simulink library "CTC_lib"  (Simulink 7.4)
settings: Solver=ode45  StartTime=0.0  StopTime=10.0  RelTol=1e-3
values from neighbouring files (symbols this model uses):
  CTCc_cnt_PrecGradVoltDeb = mpt.Parameter    [CTC_CAL.m]
  CTCc_i_HVCnctCur_max = mpt.Parameter    [CTC_CAL.m]
  CTCc_i_HVDcnctCur_max = mpt.Parameter    [CTC_CAL.m]
  CTCc_i_HVDcncWaitCur_max = mpt.Parameter    [CTC_CAL.m]
  CTCc_i_PrecCur_max = mpt.Parameter    [CTC_CAL.m]
  CTCc_pct_HVCnctTarVolt = mpt.Parameter    [CTC_CAL.m]
  CTCc_pct_HVDcnctTarVolt = mpt.Parameter    [CTC_CAL.m]
  CTCc_pct_NegCtrDiagCld = mpt.Parameter    [CTC_CAL.m]
  CTCc_pct_NegCtrDiagOpen = mpt.Parameter    [CTC_CAL.m]
  CTCc_pct_PosCtrDiagCld = mpt.Parameter    [CTC_CAL.m]
  CTCc_pct_PosCtrDiagOpen = mpt.Parameter    [CTC_CAL.m]
  CTCc_pct_PrecTarVolt = mpt.Parameter    [CTC_CAL.m]
  CTCc_pct_PrecVoltAllow = mpt.Parameter    [CTC_CAL.m]
  CTCc_tm_CtrClsCheckDly = mpt.Parameter    [CTC_CAL.m]
  CTCc_tm_CtrClsCheckDly_max = mpt.Parameter    [CTC_CAL.m]
  CTCc_tm_CtrOpenCheck_max = mpt.Parameter    [CTC_CAL.m]
  CTCc_tm_CtrOpenCheckDly = mpt.Parameter    [CTC_CAL.m]
  CTCc_tm_HVCnctTm_max = mpt.Parameter    [CTC_CAL.m]
  CTCc_tm_HVDcnctTm_max = mpt.Parameter    [CTC_CAL.m]
  CTCc_tm_HVDcnctWaitTm = mpt.Parameter    [CTC_CAL.m]
  CTCc_tm_HVDcnctWaitTm_max = mpt.Parameter    [CTC_CAL.m]
  CTCc_tm_HVEmcyDcnctTm_max = mpt.Parameter    [CTC_CAL.m]
  CTCc_tm_PrecTm_max = mpt.Parameter    [CTC_CAL.m]
  CTCc_tm_PrecVoltAlow = mpt.Parameter    [CTC_CAL.m]
  CTCc_tm_Tick_s = mpt.Parameter    [CTC_CAL.m]
  CTCc_v_PrecGradVolt = mpt.Parameter    [CTC_CAL.m]
  CTCc_v_PrecTarVoltDif = mpt.Parameter    [CTC_CAL.m]
libraries: Defined_Functionality x4
(part 2 of 2)

== stateflow chart CTC/ContactorControl ==
  settings: sampleTime=0.01
  settings: description=|
      | $Author:Zhao XiangRi$
      | $Date:2015/03/26$
      | $Revision:1.0$
  state Timer [function]
    state T1 [function]
      settings: description=$Author:Zhao XiangRi$
      state Run(Limit) [function]
        settings: description=$Author:Zhao XiangRi$
        (default) -> (junction 185)
        (junction 185) -> (junction 186) [order 1] : [Init != 1]
            | {TimeTicks = 0;TimeLimit = Limit / 10;Init = 1;}
        (junction 186) -> (junction 185)
        (junction 185) -> (junction 187) [order 2] : {TimeTicks++;}
        (junction 187) -> (junction 188) [order 1] : [TimeTicks >= TimeLimit]{Timeout = 1;}
        (junction 187) -> (junction 189) [order 2]
      state Clear [function]
        settings: description=$Author:Zhao XiangRi$
        (default) -> (junction 190)
        (junction 190) -> (junction 191) : {Timeout = 0;Init = 0;}
    state T2 [function]
      settings: description=$Author:Zhao XiangRi$
      state Run(Limit) [function]
        settings: description=$Author:Zhao XiangRi$
        (default) -> (junction 192)
        (junction 192) -> (junction 193) [order 1] : [Init != 1]{TimeTicks = 0;TimeLimit = Limit / 10;Init = 1;}
        (junction 193) -> (junction 192)
        (junction 192) -> (junction 194) [order 2] : {TimeTicks++;}
        (junction 194) -> (junction 195) [order 1] : [TimeTicks >= TimeLimit]{Timeout = 1;}
        (junction 194) -> (junction 196) [order 2]
      state Clear [function]
        settings: description=$Author:Zhao XiangRi$
        (default) -> (junction 197)
        (junction 197) -> (junction 198) : {Timeout = 0;
            | Init = 0;}
    state T3 [function]
      settings: description=$Author:Zhao XiangRi$
      state Run(Limit) [function]
        settings: description=$Author:Zhao XiangRi$
        (default) -> (junction 199)
        (junction 199) -> (junction 200) [order 1] : [Init != 1]{TimeTicks = 0;TimeLimit = Limit / 10;Init = 1;}
        (junction 200) -> (junction 199)
        (junction 199) -> (junction 201) [order 2] : {TimeTicks++;}
        (junction 201) -> (junction 202) [order 1] : [TimeTicks >= TimeLimit]{Timeout = 1;}
        (junction 201) -> (junction 203) [order 2]
      state Clear [function]
        settings: description=$Author:Zhao XiangRi$
        (default) -> (junction 204)
        (junction 204) -> (junction 205) : {Timeout = 0;Init = 0;}
    state T4 [function]
      settings: description=$Author:Zhao XiangRi$
      state Run(Limit) [function]
        settings: description=$Author:Zhao XiangRi$
        (default) -> (junction 206)
        (junction 206) -> (junction 207) [order 1] : [Init != 1]{TimeTicks = 0;TimeLimit = Limit / 10;Init = 1;}
        (junction 207) -> (junction 206)
        (junction 206) -> (junction 208) [order 2] : {TimeTicks++;}
        (junction 208) -> (junction 209) [order 1] : [TimeTicks >= TimeLimit]{Timeout = 1;}
        (junction 208) -> (junction 210) [order 2]
      state Clear [function]
        settings: description=$Author:Zhao XiangRi$
        (default) -> (junction 211)
        (junction 211) -> (junction 212) : {Timeout = 0;Init = 0;}
  state FastCharge
    settings: description=|
        | $Author:Zhao XiangRi$
        | $Date:2015/03/25$
        | $Revision:1.0$
    state FastChaCtrConnect
      en:
      CTCd_enum_CtrSt = CTC_FastChaConnect_St;
      FastChaConnectFinish=0;
      settings: description=$Author:Zhao XiangRi$
      state FastChaContactorControl
        en:
        CTCd_flg_FastChaCtrSt=0;
        ex:
        Timer.T1.Clear();
        state CloseFastChaContactorFinish
          en:
          CTCd_flg_FastChaCtrSt=1;
        state CloseFastChaContactor
          en:
          CTCd_flg_FastChaCtrReq= 1;
          du:
          Timer.T1.Run(CTCc_tm_CtrClsCheckDly);
          ex:
          Timer.T1.Clear();
        CloseFastChaContactor -> CloseFastChaContactorFinish : [Timer.T1.Timeout==1]
        (default) -> CloseFastChaContactor
      state FastChaConnectFinish
        en:
        FastChaConnectFinish=1;
      state NegContactorControl
        en:
        CTCd_flg_NegCtrSt=0;
        ex:
        Timer.T1.Clear();
        Timer.T2.Clear();
        CTCd_iflt_NegCtrStuckOpen_fault=0;
        state CloseNegContactorFinish
          en:
          CTCd_flg_NegCtrSt=1;
          CTCd_iflt_NegCtrStuckOpen_fault=0;
        state CloseNegTimeOut
          en:
          CTCd_iflt_NegCtrStuckOpen_fault=1;
        state CloseNegContactor
          en:
          CTCd_flg_NegCtrReq= 1;
          du:
          Timer.T1.Run(CTCc_tm_CtrClsCheckDly);
          Timer.T2.Run(CTCc_tm_CtrClsCheckDly_max);
        (default) -> FastCharge.FastChaCtrConnect.NegContactorControl.CloseNegContactor
        FastCharge.FastChaCtrConnect.NegContactorControl.CloseNegTimeOut -> FastCharge.FastChaCtrConnect.NegContactorControl.CloseNegContactor
        FastCharge.FastChaCtrConnect.NegContactorControl.CloseNegContactor -> FastCharge.FastChaCtrConnect.NegContactorControl.CloseNegTimeOut [order 1] : [Timer.T2.Timeout==1&&CTCd_iflt_NegCtrStuckOpen_fault!=1]
        FastCharge.FastChaCtrConnect.NegContactorControl.CloseNegContactor -> FastCharge.FastChaCtrConnect.NegContactorControl.CloseNegContactorFinish [order 2] : [UAct3 <= UAct1 *(1+ CTCc_pct_NegCtrDiagCld)&&...
            | UAct3 >= UAct1 *(1- CTCc_pct_NegCtrDiagCld)&&...
            | Timer.T1.Timeout==1]
      (default) -> FastCharge.FastChaCtrConnect.NegContactorControl
      FastCharge.FastChaCtrConnect.NegContactorControl.CloseNegContactorFinish -> FastCharge.FastChaCtrConnect.FastChaContactorControl : [CTCd_flg_NegCtrSt==1]
      CloseFastChaContactorFinish -> FastCharge.FastChaCtrConnect.FastChaConnectFinish : [CTCd_flg_FastChaCtrSt==1]
    state FastChaOffline
      CTCd_enum_CtrSt = CTC_FastChaOffline_St;
      CTCd_flg_NegCtrReq = 0;
      CTCd_flg_FastChaCtrReq = 0;
      CTCd_flg_NegCtrSt = 0;
      CTCd_flg_FastChaCtrSt = 0;
      settings: description=$Author:Zhao XiangRi$
    state FastChaDisconnect
      en:
      CTCd_enum_CtrSt=CTC_FastChaDisconnect_St;
      FastChaDisconnectFinish=0;
      settings: description=$Author:Zhao XiangRi$
      state FastChaContactorControl
        state OpenFastChaContactorFinish
          en:
          CTCd_flg_FastChaCtrSt=0;
        state OpenFastChaContactor
          en:
          CTCd_flg_FastChaCtrReq= 0;
          du:
          Timer.T1.Run(CTCc_tm_CtrOpenCheckDly);
          ex:
          Timer.T1.Clear();
        OpenFastChaContactor -> OpenFastChaContactorFinish : [Timer.T1.Timeout==1]
        (default) -> OpenFastChaContactor
      state FastChaConnectFinish
        en:
        FastChaDisconnectFinish=1;
      state NegContactorControl
        ex:
        CTCd_iflt_NegCtrStuckCld_fault=0;
        state OpenNegTimeOut
          en:
          CTCd_iflt_NegCtrStuckCld_fault=1;
        state OpenPosContactorFinish
          en:
          CTCd_flg_NegCtrSt=0;
          CTCd_iflt_NegCtrStuckCld_fault=0;
        state OpenNegContactor
          en:
          CTCd_flg_NegCtrReq= 0;
          du:
          Timer.T1.Run(CTCc_tm_CtrOpenCheckDly);
          Timer.T2.Run(CTCc_tm_CtrOpenCheck_max);
          ex:
          Timer.T1.Clear();
          Timer.T2.Clear();
        FastCharge.FastChaDisconnect.NegContactorControl.OpenNegTimeOut -> FastCharge.FastChaDisconnect.NegContactorControl.OpenNegContactor
        FastCharge.FastChaDisconnect.NegContactorControl.OpenNegContactor -> FastCharge.FastChaDisconnect.NegContactorControl.OpenPosContactorFinish [order 1] : [Timer.T1.Timeout==1&&(UAct3>= UAct1 * (1 + CTCc_pct_NegCtrDiagOpen) || ...
            | UAct3<= UAct1 * (1 - CTCc_pct_NegCtrDiagOpen))]
        (default) -> FastCharge.FastChaDisconnect.NegContactorControl.OpenNegContactor
        FastCharge.FastChaDisconnect.NegContactorControl.OpenNegContactor -> FastCharge.FastChaDisconnect.NegContactorControl.OpenNegTimeOut [order 2] : [Timer.T2.Timeout==1&&CTCd_iflt_NegCtrStuckCld_fault!=1]
      FastCharge.FastChaDisconnect.NegContactorControl.OpenPosContactorFinish -> FastCharge.FastChaDisconnect.FastChaConnectFinish : [CTCd_flg_NegCtrSt==0]
      (default) -> FastCharge.FastChaDisconnect.FastChaContactorControl
      OpenFastChaContactorFinish -> FastCharge.FastChaDisconnect.NegContactorControl : [CTCd_flg_FastChaCtrSt==0]
    state FastChaCtrOnline
      en:
      CTCd_enum_CtrSt=CTC_FastChaOnline_St;
      settings: description=$Author:Zhao XiangRi$
    (default) -> FastChaOffline
    (junction 240) -> FastChaOffline
    (junction 241) -> (junction 240)
    FastChaCtrOnline -> FastChaDisconnect : [DEMd_enum_CtrCmd==CTC_FastChaOffline_CtrCmd||...
        | DEMd_enum_CtrCmd~=CTC_FastChaOnline_CtrCmd]
    FastChaOffline -> FastChaCtrConnect : [DEMd_enum_CtrCmd==CTC_FastChaOnline_CtrCmd]
    FastCharge.FastChaCtrConnect.FastChaConnectFinish -> FastChaCtrOnline : [FastChaConnectFinish==1]
    FastCharge.FastChaDisconnect.FastChaConnectFinish -> (junction 241) : [FastChaDisconnectFinish==1]
  state Drive
    settings: description=|
        | $Author:Zhao XiangRi$
        | $Date:2015/03/20$
        | $Revision:1.0$
    state Offline
      CTCd_enum_CtrSt = CTC_DriveOffline_St;
      CTCd_flg_PosCtrReq = 0;
      CTCd_flg_NegCtrReq = 0;
      CTCd_flg_PreCtrReq = 0;
      CTCd_flg_PosCtrSt = 0;
      CTCd_flg_NegCtrSt = 0;
      CTCd_flg_PreCtrSt = 0;
      ex:
      Timer.T3.Clear();
      Timer.T4.Clear();
      settings: description=$Author:Zhao XiangRi$
      state PreChargeProhibit
        en:
        PreChargeAllow=0;
        du:
        Timer.T3.Run(CTCc_tm_PrecVoltAlow);
        ex:
        Timer.T3.Clear();
      state PreChargeAllow
        en:
        PreChargeAllow=1;
        du:
        Timer.T4.Run(CTCc_tm_PrecVoltAlow);
        ex:
        Timer.T4.Clear();
      (default) -> Drive.Offline.PreChargeProhibit
      Drive.Offline.PreChargeAllow -> Drive.Offline.PreChargeProhibit [order 1] : [UAct4>= (UAct1 * CTCc_pct_PrecVoltAllow)&&...
          | Timer.T4.Timeout ==1]
      Drive.Offline.PreChargeProhibit -> Drive.Offline.PreChargeAllow : [UAct4<(UAct1 * CTCc_pct_PrecVoltAllow)&&...
          | Timer.T3.Timeout ==1]
    state PreCharge
      en:
      CTCd_enum_CtrSt=CTC_DrivePrecharge_St;
      CTCd_flg_NegCtrSt=0;
      CTCd_flg_PreCtrSt=0;
      PreChargeFinish=0;
      du:
      CurrentGuard();
      ex:
      CTCd_iflt_NegCtrStuckOpen_fault=0;
      CTCd_iflt_PrecCurOver_fault=0;
      CTCd_iflt_PrecTmOver_fault=0;
      settings: description=$Author:Zhao XiangRi$
      state CurrentGuard [function]
        settings: description=$Author:Zhao XiangRi$
        (default) -> (junction 214)
        (junction 214) -> (junction 213) [order 3]
        (junction 214) -> (junction 215) [order 2] : [IAct<= CTCc_i_PrecCur_max && CTCd_iflt_PrecCurOver_fault != 0]
            | {CTCd_iflt_PrecCurOver_fault = 0;}
        (junction 214) -> (junction 216) [order 1] : [IAct>CTCc_i_PrecCur_max&& CTCd_iflt_PrecCurOver_fault!=1]
            | {CTCd_iflt_PrecCurOver_fault=1;}
      state NegContactorControl
        en:
        CTCd_flg_NegCtrSt=0;
        ex:
        Timer.T1.Clear();
        Timer.T2.Clear();
        CTCd_iflt_NegCtrStuckOpen_fault=0;
        settings: description=$Author:Zhao XiangRi$
        state CloseNegContactor
          en:
          CTCd_flg_NegCtrReq= 1;
          du:
          Timer.T1.Run(CTCc_tm_CtrClsCheckDly);
          Timer.T2.Run(CTCc_tm_CtrClsCheckDly_max);
        state CloseNegTimeOut
          en:
          CTCd_iflt_NegCtrStuckOpen_fault=1;
        state CloseNegContactorFinish
          en:
          CTCd_flg_NegCtrSt=1;
          CTCd_iflt_NegCtrStuckOpen_fault=0;
        (default) -> Drive.PreCharge.NegContactorControl.CloseNegContactor
        Drive.PreCharge.NegContactorControl.CloseNegContactor -> Drive.PreCharge.NegContactorControl.CloseNegTimeOut [order 1] : [Timer.T2.Timeout==1&&CTCd_iflt_NegCtrStuckOpen_fault!=1]
        Drive.PreCharge.NegContactorControl.CloseNegTimeOut -> Drive.PreCharge.NegContactorControl.CloseNegContactor
        Drive.PreCharge.NegContactorControl.CloseNegContactor -> Drive.PreCharge.NegContactorControl.CloseNegContactorFinish [order 2] : [UAct3 <= UAct1 *(1+ CTCc_pct_NegCtrDiagCld)&&...
            | UAct3 >= UAct1 *(1- CTCc_pct_NegCtrDiagCld)&&...
            | Timer.T1.Timeout==1]
      state PreContactorControl
        en:
        CTCd_flg_PreCtrSt=0;
        ex:
        Timer.T1.Clear();
        settings: description=$Author:Zhao XiangRi$
        state ClosePreContactor
          en:
          CTCd_flg_PreCtrReq= 1;
          du:
          Timer.T1.Run(CTCc_tm_CtrClsCheckDly);
          ex:
          Timer.T1.Clear();
        state ClosePreContactorFinish
          en:
          CTCd_flg_PreCtrSt=1;
        (default) -> Drive.PreCharge.PreContactorControl.ClosePreContactor
        Drive.PreCharge.PreContactorControl.ClosePreContactor -> Drive.PreCharge.PreContactorControl.ClosePreContactorFinish : [Timer.T1.Timeout==1]
      state PreChargeCheck
        du:
        Timer.T3.Run(CTCc_tm_PrecTm_max);
        ex:
        CTCd_iflt_PrecTmOver_fault= 0;
        Timer.T3.Clear();
        settings: description=$Author:Zhao XiangRi$
        state VoltageGradientCheck [function]
          settings: description=$Author:Zhao XiangRi$
          state Run(GradLimit,CountLimit) [function]
            (default) -> (junction 217)
            (junction 217) -> (junction 218) [order 1] : [GradLimitCorr == 0]
                | {GradLimitCorr = GradLimit * CTCc_tm_Tick_s;}
            (junction 218) -> (junction 217)
            (junction 217) -> (junction 219) [order 2] : {UGrad = UAct2 - UMem;}
            (junction 219) -> (junction 220) : {UMem = UAct2;}
            (junction 222) -> (junction 221) [order 1] : [Count >= CountLimit]
                | {Ok = 1;}
            (junction 220) -> (junction 222) [order 1] : [UGrad * CTCc_tm_Tick_s <= GradLimitCorr]
            (junction 222) -> (junction 223) [order 2] : {Count++;}
            (junction 220) -> (junction 223) [order 2] : {Ok = 0; Count = 0;}
          state Init [function]
            (default) -> (junction 224)
            (junction 224) -> (junction 225) : {UMem = 0; UGrad = 0; Count = 0; Ok = 0;...
                | GradLimitCorr = 0;}
        state PreChargeWait
          en:
          VoltageGradientCheck.Init();
          du:
          VoltageGradientCheck.Run(CTCc_v_PrecGradVolt,CTCc_cnt_PrecGradVoltDeb);
        state PrecDurMaxError
          en:
          CTCd_iflt_PrecTmOver_fault=1;
        state PreChargeFinish
          en:
          PreChargeFinish=1;
          CTCd_iflt_PrecTmOver_fault=0;
        (default) -> Drive.PreCharge.PreChargeCheck.PreChargeWait
        Drive.PreCharge.PreChargeCheck.PreChargeWait -> Drive.PreCharge.PreChargeCheck.PrecDurMaxError [order 2] : [Timer.T3.Timeout ==1 &&CTCd_iflt_PrecTmOver_fault!= 1]
        Drive.PreCharge.PreChargeCheck.PrecDurMaxError -> Drive.PreCharge.PreChargeCheck.PreChargeWait
        Drive.PreCharge.PreChargeCheck.PreChargeWait -> Drive.PreCharge.PreChargeCheck.PreChargeFinish [order 1] : [UAct2>= (UAct1 * CTCc_pct_PrecTarVolt)&&...
            | (UAct1 - UAct2) <= CTCc_v_PrecTarVoltDif&&...
            | VoltageGradientCheck.Ok == 1&&...
            | CTCd_flg_PreCtrSt==1&&CTCd_flg_NegCtrSt==1]
      (default) -> Drive.PreCharge.NegContactorControl
      Drive.PreCharge.NegContactorControl.CloseNegContactorFinish -> Drive.PreCharge.PreContactorControl : [CTCd_flg_NegCtrSt==1]
      Drive.PreCharge.PreContactorControl.ClosePreContactorFinish -> Drive.PreCharge.PreChargeCheck : [CTCd_flg_PreCtrSt==1]
    state Connect
      en:
      CTCd_enum_CtrSt=...
      CTC_DriveConnect_St;
      CTCd_flg_PosCtrSt=0;
      ConnectFinish=0;
      ex:
      CTCd_iflt_HVCnctCurOver_fault = 0;
      CTCd_iflt_HVCnctTmOver_fault=0;
      settings: description=$Author:Zhao XiangRi$
      state ConnectControl [parallel]
        settings: executionOrder=1  description=$Author:Zhao XiangRi$
        state PosContactorControl
          en:
          CTCd_flg_PosCtrSt=0;
          ex:
          CTCd_iflt_PosCtrStuckOpen_fault=0;
          settings: description=$Author:Zhao XiangRi$
          state ClosePosContactor
            en:
            CTCd_flg_PosCtrReq= 1;
            du:
            Timer.T1.Run(CTCc_tm_CtrClsCheckDly);
            Timer.T2.Run(CTCc_tm_CtrClsCheckDly_max);
            ex:
            Timer.T1.Clear();
            Timer.T2.Clear();
          state ClosePosTimeOut
            en:
            CTCd_iflt_PosCtrStuckOpen_fault=1;
          state ClosePosContactorFinish
            en:
            CTCd_flg_PosCtrSt=1;
            CTCd_iflt_PosCtrStuckOpen_fault=0;
          (default) -> Drive.Connect.ConnectControl.PosContactorControl.ClosePosContactor
          Drive.Connect.ConnectControl.PosContactorControl.ClosePosContactor -> Drive.Connect.ConnectControl.PosContactorControl.ClosePosTimeOut [order 1] : [Timer.T2.Timeout==1&&CTCd_iflt_PosCtrStuckOpen_fault!=1]
          Drive.Connect.ConnectControl.PosContactorControl.ClosePosTimeOut -> Drive.Connect.ConnectControl.PosContactorControl.ClosePosContactor
          Drive.Connect.ConnectControl.PosContactorControl.ClosePosContactor -> Drive.Connect.ConnectControl.PosContactorControl.ClosePosContactorFinish [order 2] : [Timer.T1.Timeout==1&&...
              | UAct2<=UAct1 * (1+CTCc_pct_PosCtrDiagCld)&& ...
              | UAct2>= UAct1 *(1-CTCc_pct_PosCtrDiagCld) ]
        state PreContactorControl
          settings: description=$Author:Zhao XiangRi$
          state OpenPreContactor
            en:
            CTCd_flg_PreCtrReq= 0;
            du:
            Timer.T1.Run(CTCc_tm_CtrOpenCheckDly);
            ex:
            Timer.T1.Clear();
          state OpenPosContactorFinish
            en:
            CTCd_flg_PreCtrSt=0;
          (default) -> Drive.Connect.ConnectControl.PreContactorControl.OpenPreContactor
          Drive.Connect.ConnectControl.PreContactorControl.OpenPreContactor -> Drive.Connect.ConnectControl.PreContactorControl.OpenPosContactorFinish : [Timer.T1.Timeout==1]
        (default) -> Drive.Connect.ConnectControl.PosContactorControl
        Drive.Connect.ConnectControl.PosContactorControl.ClosePosContactorFinish -> Drive.Connect.ConnectControl.PreContactorControl : [CTCd_flg_PosCtrSt==1]
      state ConnectCheck [parallel]
        du:
        CurrentGuard();
        Timer.T3.Run(CTCc_tm_HVCnctTm_max);
        ex:
        Timer.T3.Clear();
        settings: executionOrder=2  description=$Author:Zhao XiangRi$
        state CurrentGuard [function]
          settings: description=$Author:Zhao XiangRi$
          (default) -> (junction 227)
          (junction 227) -> (junction 226) [order 3]
          (junction 227) -> (junction 228) [order 2] : [IAct<= CTCc_i_HVCnctCur_max&& CTCd_iflt_HVCnctCurOver_fault != 0]
              | {CTCd_iflt_HVCnctCurOver_fault = 0;}
          (junction 227) -> (junction 229) [order 1] : [IAct> CTCc_i_HVCnctCur_max&& CTCd_iflt_HVCnctCurOver_fault != 1]
              | {CTCd_iflt_HVCnctCurOver_fault = 1;}
        state ConnectWait
        state CnctDurMaxError
          en:
          CTCd_iflt_HVCnctTmOver_fault=1;
        state ConnectFinish
          en:
          ConnectFinish=1;
          CTCd_iflt_HVCnctTmOver_fault=0;
        (default) -> Drive.Connect.ConnectCheck.ConnectWait
        Drive.Connect.ConnectCheck.ConnectWait -> Drive.Connect.ConnectCheck.CnctDurMaxError [order 2] : [Timer.T3.Timeout ==1&&CTCd_iflt_HVCnctTmOver_fault!=1]
        Drive.Connect.ConnectCheck.CnctDurMaxError -> Drive.Connect.ConnectCheck.ConnectWait
        Drive.Connect.ConnectCheck.ConnectWait -> Drive.Connect.ConnectCheck.ConnectFinish [order 1] : [UAct2 >= (UAct1 * CTCc_pct_HVCnctTarVolt)&&...
            |  CTCd_flg_PosCtrSt==1&&...
            | CTCd_flg_PreCtrSt==0]
    state Online
      en:
      CTCd_enum_CtrSt=CTC_DriveOnline_St;
      settings: description=$Author:Zhao XiangRi$
      state NegContactorDiagnose [parallel]
        ex:
        Timer.T1.Clear();
        CTCd_iflt_NegCtrStuckOpen_fault=0;
        settings: executionOrder=1  description=$Author:Zhao XiangRi$
        state NegContactorCheck
          en:
          CTCd_iflt_NegCtrStuckOpen_fault=0;
          Timer.T1.Clear();
        state NegContactorDiag
          du:
          Timer.T1.Run(CTCc_tm_CtrOpenCheck_max);
        state NegContactorFault
          en:
          CTCd_flg_NegCtrSt=0;
          CTCd_iflt_NegCtrStuckOpen_fault=1;
          Timer.T1.Clear();
        (default) -> Drive.Online.NegContactorDiagnose.NegContactorCheck
        Drive.Online.NegContactorDiagnose.NegContactorCheck -> Drive.Online.NegContactorDiagnose.NegContactorDiag : [UAct3 > UAct1 *(1+ CTCc_pct_NegCtrDiagOpen)||...
            | UAct3 < UAct1 *(1- CTCc_pct_NegCtrDiagOpen)]
        Drive.Online.NegContactorDiagnose.NegContactorDiag -> Drive.Online.NegContactorDiagnose.NegContactorCheck [order 1] : [UAct3 < UAct1 *(1+ CTCc_pct_NegCtrDiagCld)&&...
            | UAct3 >UAct1 *(1- CTCc_pct_NegCtrDiagCld)]
        Drive.Online.NegContactorDiagnose.NegContactorDiag -> Drive.Online.NegContactorDiagnose.NegContactorFault [order 2] : [(UAct3 > UAct1 *(1+ CTCc_pct_NegCtrDiagOpen)||...
            | UAct3 < UAct1 *(1- CTCc_pct_NegCtrDiagOpen))&&...
            | (CTCd_iflt_NegCtrStuckOpen_fault!=1)&&...
            | Timer.T1.Timeout==1]
      state PosContactorDiagnose [parallel]
        ex:
        Timer.T2.Clear();
        CTCd_iflt_PosCtrStuckOpen_fault=0;
        settings: executionOrder=2  description=$Author:Zhao XiangRi$
        state PosContactorDiag
          du:
          Timer.T2.Run(CTCc_tm_CtrOpenCheck_max);
        state PosContactorCheck
          en:
          CTCd_iflt_PosCtrStuckOpen_fault=0;
          Timer.T2.Clear();
        state PosContactorFault
          en:
          CTCd_flg_PosCtrSt=0;
          CTCd_iflt_PosCtrStuckOpen_fault=1;
          Timer.T2.Clear();
        (default) -> Drive.Online.PosContactorDiagnose.PosContactorCheck
        Drive.Online.PosContactorDiagnose.PosContactorCheck -> Drive.Online.PosContactorDiagnose.PosContactorDiag : [UAct2 > UAct1 *(1+ CTCc_pct_PosCtrDiagOpen)||...
            | UAct2 < UAct1 *(1- CTCc_pct_PosCtrDiagOpen)]
        Drive.Online.PosContactorDiagnose.PosContactorDiag -> Drive.Online.PosContactorDiagnose.PosContactorCheck [order 1] : [UAct2<UAct1 *(1+ CTCc_pct_PosCtrDiagCld)&&...
            | UAct2>UAct1 *(1- CTCc_pct_PosCtrDiagCld)]
        Drive.Online.PosContactorDiagnose.PosContactorDiag -> Drive.Online.PosContactorDiagnose.PosContactorFault [order 2] : [(UAct2 > UAct1 *(1+ CTCc_pct_PosCtrDiagOpen)||...
            | UAct2 < UAct1 *(1- CTCc_pct_PosCtrDiagOpen))&&...
            | CTCd_iflt_PosCtrStuckOpen_fault!=1&&...
            | Timer.T2.Timeout==1]
    state EmergencyDisconnect
      en:
      CTCd_enum_CtrSt=...
      CTC_DriveEmgyDcnct_St;
      DcnctEmcyFinish = 0;
      settings: description=$Author:Zhao XiangRi$
      state EmcyDisconnectControl [parallel]
        en:
        CTCd_flg_PosCtrReq= 0;
        CTCd_flg_NegCtrReq= 0;
        CTCd_flg_PreCtrReq= 0;
        DcnctEmcyCtlFinish = 1;
        settings: executionOrder=1  description=$Author:Zhao XiangRi$
      state EmcyDisconnectCheck [parallel]
        du:
        Timer.T1.Run(CTCc_tm_HVEmcyDcnctTm_max);
        ex:
        Timer.T1.Clear();
        settings: executionOrder=2  description=$Author:Zhao XiangRi$
        state DisconnectWait
        state DisconnectComplete
          DcnctEmcyFinish = 1;
        state DisconnectTimeoutError
          en:
          CTCd_iflt_HVEmcyDcnctTmOver_fault = 1;
          ex:
          CTCd_iflt_HVEmcyDcnctTmOver_fault = 0;
        (default) -> Drive.EmergencyDisconnect.EmcyDisconnectCheck.DisconnectWait
        Drive.EmergencyDisconnect.EmcyDisconnectCheck.DisconnectWait -> Drive.EmergencyDisconnect.EmcyDisconnectCheck.DisconnectComplete [order 2] : [DcnctEmcyCtlFinish==1 &&IAct<= CTCc_i_HVDcnctCur_max &&...
            | (UAct2>= UAct1 * (1 + CTCc_pct_HVDcnctTarVolt) ||UAct2<= UAct1 * (1 - CTCc_pct_HVDcnctTarVolt))]
            | {CTCd_flg_PosCtrSt=0;CTCd_flg_NegCtrSt=0;CTCd_flg_PreCtrSt=0;}
        Drive.EmergencyDisconnect.EmcyDisconnectCheck.DisconnectWait -> Drive.EmergencyDisconnect.EmcyDisconnectCheck.DisconnectTimeoutError [order 1] : [Timer.T1.Timeout == 1]
        Drive.EmergencyDisconnect.EmcyDisconnectCheck.DisconnectTimeoutError -> Drive.EmergencyDisconnect.EmcyDisconnectCheck.DisconnectComplete : [DcnctEmcyCtlFinish==1 &&...
            | (UAct2>= UAct1 * (1 +CTCc_pct_HVDcnctTarVolt) ||UAct2<= UAct1 * (1 - CTCc_pct_HVDcnctTarVolt))]
            | {CTCd_flg_PosCtrSt=0;CTCd_flg_NegCtrSt=0;CTCd_flg_PreCtrSt=0;}
    state Shutoff
      en:
      CTCd_enum_CtrSt=CTC_DriveShutoff_St;
      ShutoffFinish=0;
      ex:
      CTCd_iflt_HVDcncWaitTmOver_fault=0;
      Timer.T1.Clear();
      Timer.T2.Clear();
      settings: description=$Author:Zhao XiangRi$
      state ShutoffDelay
        en:
        ShutoffFinish = 0;
        du:
        Timer.T1.Run(CTCc_tm_HVDcnctWaitTm_max);
        Timer.T2.Run(CTCc_tm_HVDcnctWaitTm);
      state SoffDurMaxError
        en:
        CTCd_iflt_HVDcncWaitTmOver_fault = 1;
      state ShutoffComplete
        en:
        ShutoffFinish=1;
        CTCd_iflt_HVDcncWaitTmOver_fault = 0;
      (default) -> ShutoffDelay
      ShutoffDelay -> SoffDurMaxError [order 2] : [Timer.T1.Timeout == 1 && CTCd_iflt_HVDcncWaitTmOver_fault != 1]
      SoffDurMaxError -> ShutoffDelay
      ShutoffDelay -> ShutoffComplete [order 1] : [Timer.T2.Timeout == 1&&IAct<= CTCc_i_HVDcncWaitCur_max]
    state Disconnect
      en:
      CTCd_enum_CtrSt=...
      CTC_DriveDisconnect_St;
      DisConnectFinish=0;
      ex:
      CTCd_iflt_HVDcnctTmOver_fault = 0;
      settings: description=$Author:Zhao XiangRi$
      state DisconnectControl [parallel]
        settings: executionOrder=1  description=$Author:Zhao XiangRi$
        state PosContactorControl
          ex:
          CTCd_iflt_PosCtrStuckCld_fault=0;
          settings: description=$Author:Zhao XiangRi$
          state OpenPosContactor
            en:
            CTCd_flg_PosCtrReq= 0;
            du:
            Timer.T1.Run(CTCc_tm_CtrOpenCheckDly);
            Timer.T2.Run(CTCc_tm_CtrOpenCheck_max);
            ex:
            Timer.T1.Clear();
            Timer.T2.Clear();
          state OpenPosTimeOut
            en:
            CTCd_iflt_PosCtrStuckCld_fault=1;
          state OpenPosContactorFinish
            en:
            CTCd_flg_PosCtrSt=0;
            CTCd_iflt_PosCtrStuckCld_fault=0;
          (default) -> Drive.Disconnect.DisconnectControl.PosContactorControl.OpenPosContactor
          Drive.Disconnect.DisconnectControl.PosContactorControl.OpenPosContactor -> Drive.Disconnect.DisconnectControl.PosContactorControl.OpenPosTimeOut [order 1] : [Timer.T2.Timeout==1&&CTCd_iflt_PosCtrStuckCld_fault!=1]
          Drive.Disconnect.DisconnectControl.PosContactorControl.OpenPosTimeOut -> Drive.Disconnect.DisconnectControl.PosContactorControl.OpenPosContactor
          Drive.Disconnect.DisconnectControl.PosContactorControl.OpenPosContactor -> Drive.Disconnect.DisconnectControl.PosContactorControl.OpenPosContactorFinish [order 2] : [Timer.T1.Timeout==1&&(UAct2>= UAct1 * (1 + CTCc_pct_PosCtrDiagOpen) || ...
              | UAct2<= UAct1 * (1 - CTCc_pct_PosCtrDiagOpen))]
        state NegContactorControl
          ex:
          CTCd_iflt_NegCtrStuckCld_fault=0;
          settings: description=$Author:Zhao XiangRi$
          state OpenNegContactor
            en:
            CTCd_flg_NegCtrReq= 0;
            du:
            Timer.T1.Run(CTCc_tm_CtrOpenCheckDly);
            Timer.T2.Run(CTCc_tm_CtrOpenCheck_max);
            ex:
            Timer.T1.Clear();
            Timer.T2.Clear();
          state OpenNegTimeOut
            en:
            CTCd_iflt_NegCtrStuckCld_fault=1;
          state OpenPosContactorFinish
            en:
            CTCd_flg_NegCtrSt=0;
            CTCd_iflt_NegCtrStuckCld_fault=0;
          (default) -> Drive.Disconnect.DisconnectControl.NegContactorControl.OpenNegContactor
          Drive.Disconnect.DisconnectControl.NegContactorControl.OpenNegContactor -> Drive.Disconnect.DisconnectControl.NegContactorControl.OpenNegTimeOut [order 2] : [Timer.T2.Timeout==1&&CTCd_iflt_NegCtrStuckCld_fault!=1]
          Drive.Disconnect.DisconnectControl.NegContactorControl.OpenNegTimeOut -> Drive.Disconnect.DisconnectControl.NegContactorControl.OpenNegContactor
          Drive.Disconnect.DisconnectControl.NegContactorControl.OpenNegContactor -> Drive.Disconnect.DisconnectControl.NegContactorControl.OpenPosContactorFinish [order 1] : [Timer.T1.Timeout==1&&(UAct3>= UAct1 * (1 + CTCc_pct_NegCtrDiagOpen) || ...
              | UAct3<= UAct1 * (1 - CTCc_pct_NegCtrDiagOpen))]
        (default) -> Drive.Disconnect.DisconnectControl.PosContactorControl
        Drive.Disconnect.DisconnectControl.PosContactorControl.OpenPosContactorFinish -> Drive.Disconnect.DisconnectControl.NegContactorControl : [CTCd_flg_PosCtrSt==0]
      state DisConnectCheck [parallel]
        du:
        Timer.T3.Run(CTCc_tm_HVDcnctTm_max);
        ex:
        Timer.T3.Clear();
        settings: executionOrder=2  description=$Author:Zhao XiangRi$
        state CnctDurMaxError
          en:
          CTCd_iflt_HVDcnctTmOver_fault = 1;
        state DisConnectWait
        state DisConnectFinish
          en:
          DisConnectFinish=1;
          CTCd_iflt_HVDcnctTmOver_fault=0;
        (default) -> Drive.Disconnect.DisConnectCheck.DisConnectWait
        Drive.Disconnect.DisConnectCheck.DisConnectWait -> Drive.Disconnect.DisConnectCheck.CnctDurMaxError [order 1] : [Timer.T3.Timeout ==1&& CTCd_iflt_HVDcnctTmOver_fault != 1]
        Drive.Disconnect.DisConnectCheck.CnctDurMaxError -> Drive.Disconnect.DisConnectCheck.DisConnectWait
        Drive.Disconnect.DisConnectCheck.DisConnectWait -> Drive.Disconnect.DisConnectCheck.DisConnectFinish [order 2] : [(UAct2<= UAct1 * (1 - CTCc_pct_HVDcnctTarVolt)||...
            | UAct2>= UAct1 * (1 + CTCc_pct_HVDcnctTarVolt) )&& ...
            | IAct<CTCc_i_HVDcnctCur_max&&...
            | CTCd_flg_PosCtrSt==0&&CTCd_flg_NegCtrSt==0]
    (default) -> Drive.Offline
    (junction 230) -> Drive.Offline
    (junction 231) -> Drive.Offline
    (junction 236) -> (junction 231)
    Drive.PreCharge -> (junction 232) : [DEMd_enum_CtrCmd==CTC_DriveEmgyDcnct_CtrCmd||...
        | CTCd_iflt_NegCtrStuckOpen_fault==1||...
        | CTCd_iflt_PrecCurOver_fault==1||...
        | CTCd_iflt_PrecTmOver_fault==1]
    (junction 232) -> (junction 233)
    Drive.Connect -> (junction 233) : [DEMd_enum_CtrCmd==CTC_DriveEmgyDcnct_CtrCmd||...
        | CTCd_iflt_HVCnctCurOver_fault==1||...
        | CTCd_iflt_HVCnctTmOver_fault==1]
    (junction 233) -> (junction 234)
    Drive.Online -> (junction 234) [order 1] : [DEMd_enum_CtrCmd==CTC_DriveEmgyDcnct_CtrCmd]
    (junction 234) -> Drive.EmergencyDisconnect
    (junction 235) -> (junction 234)
    Shutoff -> Drive.Online [order 2] : [DEMd_enum_CtrCmd==...
        | CTC_DriveOnline_CtrCmd]
    Drive.Online -> Shutoff [order 2] : [(DEMd_enum_CtrCmd==CTC_DriveOffline_CtrCmd)||...
        | (DEMd_enum_CtrCmd~=CTC_DriveOnline_CtrCmd...
        | &&DEMd_enum_CtrCmd~=CTC_DriveEmgyDcnct_CtrCmd)]
    Shutoff -> (junction 235) [order 1] : [DEMd_enum_CtrCmd==CTC_DriveEmgyDcnct_CtrCmd||...
        | CTCd_iflt_HVDcncWaitTmOver_fault==1]
    (junction 237) -> (junction 235)
    Drive.Disconnect -> (junction 237) : [DEMd_enum_CtrCmd==CTC_DriveEmgyDcnct_CtrCmd||...
        | CTCd_iflt_HVDcnctTmOver_fault==1]
    Drive.Offline.PreChargeAllow -> Drive.PreCharge [order 2] : [DEMd_enum_CtrCmd==CTC_DriveOnline_CtrCmd&&...
        | BSCd_enum_BCUSt==BCU_Drive_St&&...
        | PreChargeAllow==1]
    Drive.PreCharge.PreChargeCheck.PreChargeFinish -> Drive.Connect : [PreChargeFinish==1]
    Drive.Connect.ConnectCheck.ConnectFinish -> Drive.Online : [ConnectFinish==1]
    ShutoffComplete -> Drive.Disconnect : [ShutoffFinish==1]
    Drive.EmergencyDisconnect.EmcyDisconnectCheck.DisconnectComplete -> (junction 230) : [DcnctEmcyFinish == 1]
    Drive.Disconnect.DisConnectCheck.DisConnectFinish -> (junction 236) : [DisConnectFinish==1]
  state Service
    settings: description=|
        | $Author:Zhao XiangRi$
        | $Date:2015/03/27$
        | $Revision:1.0$
    state ServiceOffline
      CTCd_enum_CtrSt = CTC_ServiceOffline_St;
      CTCd_flg_PosCtrReq = 0;
      CTCd_flg_NegCtrReq = 0;
      CTCd_flg_PreCtrReq = 0;
      CTCd_flg_FastChaCtrReq = 0;
      CTCd_flg_SlowChaCtrReq = 0;
      CTCd_flg_PosCtrSt = 0;
      CTCd_flg_NegCtrSt = 0;
      CTCd_flg_PreCtrSt = 0;
      CTCd_flg_FastChaCtrSt = 0;
      CTCd_flg_SlowChaCtrSt = 0;
    state NegContactorControl
      en:
      CTCd_enum_CtrSt = CTC_ServiceOnline_St;;
      settings: description=$Author:Zhao XiangRi$
      state CloseNegCtr
        en:
        CTCd_flg_NegCtrReq= 1;
        du:
        Timer.T1.Run(CTCc_tm_CtrClsCheckDly_max);
        ex:
        Timer.T1.Clear();
        CloseNegCtr -> CloseNegCtr [order 1] : [Timer.T1.Timeout==1 &&...
            | UAct3 <= UAct1 *(1+ CTCc_pct_NegCtrDiagCld)&&...
            | UAct3 >= UAct1 *(1- CTCc_pct_NegCtrDiagCld)]
            | {CTCd_flg_NegCtrSt=1;}
      state OpenNegCtr
        en:
        CTCd_flg_NegCtrReq= 0;
        du:
        Timer.T2.Run(CTCc_tm_CtrOpenCheck_max);
        ex:
        Timer.T2.Clear();
        OpenNegCtr -> OpenNegCtr : [Timer.T2.Timeout==1 && ...
            | UAct3>= UAct1 * (1 + CTCc_pct_NegCtrDiagOpen) || ...
            | UAct3<= UAct1 * (1 - CTCc_pct_NegCtrDiagOpen)]
            | {CTCd_flg_NegCtrSt=0;Lock=0;}
      (default) -> CloseNegCtr
      CloseNegCtr -> OpenNegCtr [order 1] : [IPTd_enum_ServCmd ==CTC_OpenNegCtr_SerCmd || ...
          | IPTd_enum_ServCmd !=CTC_CloseNegCtr_SerCmd||...
          | BSCd_enum_BCUSt!=BCU_Service_St]
    state PosContactorControl
      en:
      CTCd_enum_CtrSt = CTC_ServiceOnline_St;;
      settings: description=$Author:Zhao XiangRi$
      state ClosePosCtr
        en:
        CTCd_flg_PosCtrReq= 1;
        du:
        Timer.T1.Run(CTCc_tm_CtrClsCheckDly_max);
        ex:
        Timer.T1.Clear();
        ClosePosCtr -> ClosePosCtr [order 1] : [Timer.T1.Timeout==1 &&...
            | UAct2<=UAct1 * (1+CTCc_pct_PosCtrDiagCld)&& ...
            | UAct2>= UAct1 *(1+-CTCc_pct_PosCtrDiagCld)]
            | {CTCd_flg_PosCtrSt=1;}
      state OpenPosCtr
        en:
        CTCd_flg_PosCtrReq= 0;
        du:
        Timer.T2.Run(CTCc_tm_CtrOpenCheck_max);
        ex:
        Timer.T2.Clear();
        OpenPosCtr -> OpenPosCtr : [Timer.T2.Timeout==1 && ...
            | UAct2>= UAct1 * (1 + CTCc_pct_PosCtrDiagOpen) || ...
            | UAct2<= UAct1 * (1 - CTCc_pct_PosCtrDiagOpen)]
            | {CTCd_flg_PosCtrSt=0;Lock=0;}
      ClosePosCtr -> OpenPosCtr [order 1] : [IPTd_enum_ServCmd ==CTC_OpenPosCtr_SerCmd || ...
          | IPTd_enum_ServCmd !=CTC_ClosePosCtr_SerCmd||...
          | BSCd_enum_BCUSt!=BCU_Service_St]
      (default) -> ClosePosCtr
    state PreContactorControl
      en:
      CTCd_enum_CtrSt = CTC_ServiceOnline_St;;
      settings: description=$Author:Zhao XiangRi$
      state ClosePreCtr
        en:
        CTCd_flg_PreCtrReq= 1;
        du:
        Timer.T1.Run(CTCc_tm_CtrClsCheckDly_max);
        ex:
        Timer.T1.Clear();
        ClosePreCtr -> ClosePreCtr [order 1] : [Timer.T1.Timeout==1 &&...
            | UAct2<=UAct1 * (1+CTCc_pct_PosCtrDiagCld)&& ...
            | UAct2>= UAct1 *(1+-CTCc_pct_PosCtrDiagCld)&&...
            |  CTCd_flg_PreCtrSt != 1]
            | {CTCd_flg_PreCtrSt=1;}
      state OpenPreCtr
        en:
        CTCd_flg_PreCtrReq= 0;
        du:
        Timer.T2.Run(CTCc_tm_CtrOpenCheck_max);
        ex:
        Timer.T2.Clear();
        OpenPreCtr -> OpenPreCtr : [Timer.T2.Timeout==1 && ...
            | UAct2>= UAct1 * (1 + CTCc_pct_PosCtrDiagOpen) || ...
            | UAct2<= UAct1 * (1 - CTCc_pct_PosCtrDiagOpen)]
            | {CTCd_flg_PreCtrSt=0;Lock=0;}
      ClosePreCtr -> OpenPreCtr [order 1] : [IPTd_enum_ServCmd ==CTC_OpenPreCtr_SerCmd || ...
          | IPTd_enum_ServCmd !=CTC_ClosePreCtr_SerCmd||...
          | BSCd_enum_BCUSt!=BCU_Service_St]
      (default) -> ClosePreCtr
    state FastChaContactorControl
      en:
      CTCd_enum_CtrSt = CTC_ServiceOnline_St;;
      settings: description=$Author:Zhao XiangRi$
      state CloseFastChaCtr
        en:
        CTCd_flg_FastChaCtrReq= 1;
        du:
        Timer.T1.Run(CTCc_tm_CtrClsCheckDly_max);
        ex:
        Timer.T1.Clear();
        CloseFastChaCtr -> CloseFastChaCtr [order 1] : [Timer.T1.Timeout==1]
            | {CTCd_flg_FastChaCtrSt=1;}
      state OpenFastChaNegCtr
        en:
        CTCd_flg_FastChaCtrReq= 0;
        du:
        Timer.T2.Run(CTCc_tm_CtrOpenCheck_max);
        ex:
        Timer.T2.Clear();
        OpenFastChaNegCtr -> OpenFastChaNegCtr : [Timer.T2.Timeout==1]
            | {CTCd_flg_FastChaCtrSt=0;Lock=0;}
      CloseFastChaCtr -> OpenFastChaNegCtr [order 1] : [IPTd_enum_ServCmd ==CTC_OpenFastChaCtr_SerCmd || ...
          | IPTd_enum_ServCmd !=CTC_CloseFastChaCtr_SerCmd||...
          | BSCd_enum_BCUSt!=BCU_Service_St]
      (default) -> CloseFastChaCtr
    state SlowChaContactorControl
      en:
      CTCd_enum_CtrSt = CTC_ServiceOnline_St;;
      settings: description=$Author:Zhao XiangRi$
      state CloseSlowChaCtr
        en:
        CTCd_flg_SlowChaCtrReq= 1;
        du:
        Timer.T1.Run(CTCc_tm_CtrClsCheckDly_max);
        ex:
        Timer.T1.Clear();
        CloseSlowChaCtr -> CloseSlowChaCtr [order 1] : [Timer.T1.Timeout==1]
            | {CTCd_flg_SlowChaCtrSt=1;}
      state OpenSlowChaCtr
        en:
        CTCd_flg_SlowChaCtrReq= 0;
        du:
        Timer.T2.Run(CTCc_tm_CtrOpenCheck_max);
        ex:
        Timer.T2.Clear();
        OpenSlowChaCtr -> OpenSlowChaCtr : [Timer.T2.Timeout==1]
            | {CTCd_flg_SlowChaCtrSt=0;Lock=0;}
      CloseSlowChaCtr -> OpenSlowChaCtr [order 1] : [IPTd_enum_ServCmd ==CTC_OpenSlowChaCtr_SerCmd || ...
          | IPTd_enum_ServCmd !=CTC_CloseSlowChaCtr_SerCmd||...
          | BSCd_enum_BCUSt!=BCU_Service_St]
      (default) -> CloseSlowChaCtr
    Service.NegContactorControl -> ServiceOffline : [CTCd_flg_NegCtrSt==0&&Lock==0]
    ServiceOffline -> Service.NegContactorControl [order 2] : [IPTd_enum_ServCmd ==...
        | CTC_CloseNegCtr_SerCmd]{Lock=1;}
    (default) -> ServiceOffline
    ServiceOffline -> Service.PosContactorControl [order 4] : [IPTd_enum_ServCmd ==...
        | CTC_ClosePosCtr_SerCmd]{Lock=1;}
    Service.PosContactorControl -> ServiceOffline : [CTCd_flg_PosCtrSt==0&&Lock==0]
    ServiceOffline -> Service.PreContactorControl [order 5] : [IPTd_enum_ServCmd ==...
        | CTC_ClosePreCtr_SerCmd]{Lock=1;}
    Service.PreContactorControl -> ServiceOffline : [CTCd_flg_PreCtrSt==0&&Lock==0]
    ServiceOffline -> Service.FastChaContactorControl [order 3] : [IPTd_enum_ServCmd ==...
        | CTC_CloseFastChaCtr_SerCmd]{Lock=1;}
    Service.FastChaContactorControl -> ServiceOffline : [CTCd_flg_FastChaCtrSt==0&&Lock==0]
    ServiceOffline -> SlowChaContactorControl [order 1] : [IPTd_enum_ServCmd ==...
        | CTC_CloseSlowChaCtr_SerCmd]{Lock=1;}
    SlowChaContactorControl -> ServiceOffline : [CTCd_flg_SlowChaCtrSt==0&&Lock==0]
  state DefaultOffline
    CTCd_enum_CtrSt=CTC_DefaultOffline_St;
    CTCd_flg_PosCtrReq = 0;
    CTCd_flg_NegCtrReq = 0;
    CTCd_flg_PreCtrReq = 0;
    CTCd_flg_FastChaCtrReq = 0;
    CTCd_flg_SlowChaCtrReq = 0;
    CTCd_flg_PosCtrSt = 0;
    CTCd_flg_NegCtrSt = 0;
    CTCd_flg_PreCtrSt = 0;
    CTCd_flg_FastChaCtrSt = 0;
    CTCd_flg_SlowChaCtrSt = 0;
  state SlowCharge
    settings: description=|
        | $Author:Zhao XiangRi$
        | $Date:2015/03/20$
        | $Revision:1.0$
    state Disconnect
      en:
      CTCd_enum_CtrSt=...
      CTC_SlowChaDisconnect_St;
      DisConnectFinish=0;
      ex:
      CTCd_iflt_HVDcnctTmOver_fault = 0;
      settings: description=$Author:Zhao XiangRi$
      state DisConnectCheck [parallel]
        du:
        Timer.T3.Run(CTCc_tm_HVDcnctTm_max);
        ex:
        Timer.T3.Clear();
        settings: executionOrder=2  description=$Author:Zhao XiangRi$
        state DisConnectWait
        state CnctDurMaxError
          en:
          CTCd_iflt_HVDcnctTmOver_fault = 1;
        state DisConnectFinish
          en:
          DisConnectFinish=1;
          CTCd_iflt_HVDcnctTmOver_fault=0;
        (default) -> SlowCharge.Disconnect.DisConnectCheck.DisConnectWait
        SlowCharge.Disconnect.DisConnectCheck.DisConnectWait -> SlowCharge.Disconnect.DisConnectCheck.CnctDurMaxError [order 1] : [Timer.T3.Timeout ==1&& CTCd_iflt_HVDcnctTmOver_fault != 1]
        SlowCharge.Disconnect.DisConnectCheck.CnctDurMaxError -> SlowCharge.Disconnect.DisConnectCheck.DisConnectWait
        SlowCharge.Disconnect.DisConnectCheck.DisConnectWait -> SlowCharge.Disconnect.DisConnectCheck.DisConnectFinish [order 2] : [(UAct2<= UAct1 * (1 - CTCc_pct_HVDcnctTarVolt)||...
            | UAct2>= UAct1 * (1 + CTCc_pct_HVDcnctTarVolt) )&& ...
            | IAct<CTCc_i_HVDcnctCur_max&&...
            | CTCd_flg_PosCtrSt==0&&CTCd_flg_NegCtrSt==0]
      state DisconnectControl [parallel]
        settings: executionOrder=1  description=$Author:Zhao XiangRi$
        state NegContactorControl
          ex:
          CTCd_iflt_NegCtrStuckCld_fault=0;
          settings: description=$Author:Zhao XiangRi$
          state OpenPosContactorFinish
            en:
            CTCd_flg_NegCtrSt=0;
            CTCd_iflt_NegCtrStuckCld_fault=0;
          state OpenNegTimeOut
            en:
            CTCd_iflt_NegCtrStuckCld_fault=1;
          state OpenNegContactor
            en:
            CTCd_flg_NegCtrReq= 0;
            du:
            Timer.T1.Run(CTCc_tm_CtrOpenCheckDly);
            Timer.T2.Run(CTCc_tm_CtrOpenCheck_max);
            ex:
            Timer.T1.Clear();
            Timer.T2.Clear();
          SlowCharge.Disconnect.DisconnectControl.NegContactorControl.OpenNegContactor -> SlowCharge.Disconnect.DisconnectControl.NegContactorControl.OpenPosContactorFinish [order 1] : [Timer.T1.Timeout==1&&(UAct3>= UAct1 * (1 + CTCc_pct_NegCtrDiagOpen) || ...
              | UAct3<= UAct1 * (1 - CTCc_pct_NegCtrDiagOpen))]
          (default) -> SlowCharge.Disconnect.DisconnectControl.NegContactorControl.OpenNegContactor
          SlowCharge.Disconnect.DisconnectControl.NegContactorControl.OpenNegContactor -> SlowCharge.Disconnect.DisconnectControl.NegContactorControl.OpenNegTimeOut [order 2] : [Timer.T2.Timeout==1&&CTCd_iflt_NegCtrStuckCld_fault!=1]
          SlowCharge.Disconnect.DisconnectControl.NegContactorControl.OpenNegTimeOut -> SlowCharge.Disconnect.DisconnectControl.NegContactorControl.OpenNegContactor
        state PosContactorControl
          ex:
          CTCd_iflt_PosCtrStuckCld_fault=0;
          settings: description=$Author:Zhao XiangRi$
          state OpenPosContactorFinish
            en:
            CTCd_flg_PosCtrSt=0;
            CTCd_iflt_PosCtrStuckCld_fault=0;
          state OpenPosTimeOut
            en:
            CTCd_iflt_PosCtrStuckCld_fault=1;
          state OpenPosContactor
            en:
            CTCd_flg_PosCtrReq= 0;
            du:
            Timer.T1.Run(CTCc_tm_CtrOpenCheckDly);
            Timer.T2.Run(CTCc_tm_CtrOpenCheck_max);
            ex:
            Timer.T1.Clear();
            Timer.T2.Clear();
          SlowCharge.Disconnect.DisconnectControl.PosContactorControl.OpenPosTimeOut -> SlowCharge.Disconnect.DisconnectControl.PosContactorControl.OpenPosContactor
          SlowCharge.Disconnect.DisconnectControl.PosContactorControl.OpenPosContactor -> SlowCharge.Disconnect.DisconnectControl.PosContactorControl.OpenPosTimeOut [order 1] : [Timer.T2.Timeout==1&&CTCd_iflt_PosCtrStuckCld_fault!=1]
          (default) -> SlowCharge.Disconnect.DisconnectControl.PosContactorControl.OpenPosContactor
          SlowCharge.Disconnect.DisconnectControl.PosContactorControl.OpenPosContactor -> SlowCharge.Disconnect.DisconnectControl.PosContactorControl.OpenPosContactorFinish [order 2] : [Timer.T1.Timeout==1&&(UAct2>= UAct1 * (1 + CTCc_pct_PosCtrDiagOpen) || ...
              | UAct2<= UAct1 * (1 - CTCc_pct_PosCtrDiagOpen))]
        (default) -> SlowCharge.Disconnect.DisconnectControl.PosContactorControl
        SlowCharge.Disconnect.DisconnectControl.PosContactorControl.OpenPosContactorFinish -> SlowCharge.Disconnect.DisconnectControl.NegContactorControl : [CTCd_flg_PosCtrSt==0]
    state Online
      en:
      CTCd_enum_CtrSt=CTC_SlowChaOnline_St;
      settings: description=$Author:Zhao XiangRi$
      state PosContactorDiagnose [parallel]
        ex:
        Timer.T2.Clear();
        CTCd_iflt_PosCtrStuckOpen_fault=0;
        settings: executionOrder=2  description=$Author:Zhao XiangRi$
        state PosContactorFault
          en:
          CTCd_flg_PosCtrSt=0;
          CTCd_iflt_PosCtrStuckOpen_fault=1;
          Timer.T2.Clear();
        state PosContactorCheck
          en:
          CTCd_iflt_PosCtrStuckOpen_fault=0;
          Timer.T2.Clear();
        state PosContactorDiag
          du:
          Timer.T2.Run(CTCc_tm_CtrOpenCheck_max);
        SlowCharge.Online.PosContactorDiagnose.PosContactorDiag -> SlowCharge.Online.PosContactorDiagnose.PosContactorFault [order 2] : [(UAct2 > UAct1 *(1+ CTCc_pct_PosCtrDiagOpen)||...
            | UAct2 < UAct1 *(1- CTCc_pct_PosCtrDiagOpen))&&...
            | CTCd_iflt_PosCtrStuckOpen_fault!=1&&...
            | Timer.T2.Timeout==1]
        SlowCharge.Online.PosContactorDiagnose.PosContactorCheck -> SlowCharge.Online.PosContactorDiagnose.PosContactorDiag : [UAct2 > UAct1 *(1+ CTCc_pct_PosCtrDiagOpen)||...
            | UAct2 < UAct1 *(1- CTCc_pct_PosCtrDiagOpen)]
        SlowCharge.Online.PosContactorDiagnose.PosContactorDiag -> SlowCharge.Online.PosContactorDiagnose.PosContactorCheck [order 1] : [UAct2<UAct1 *(1+ CTCc_pct_PosCtrDiagCld)&&...
            | UAct2>UAct1 *(1- CTCc_pct_PosCtrDiagCld)]
        (default) -> SlowCharge.Online.PosContactorDiagnose.PosContactorCheck
      state NegContactorDiagnose [parallel]
        ex:
        Timer.T1.Clear();
        CTCd_iflt_NegCtrStuckOpen_fault=0;
        settings: executionOrder=1  description=$Author:Zhao XiangRi$
        state NegContactorFault
          en:
          CTCd_flg_NegCtrSt=0;
          CTCd_iflt_NegCtrStuckOpen_fault=1;
          Timer.T1.Clear();
        state NegContactorDiag
          du:
          Timer.T1.Run(CTCc_tm_CtrOpenCheck_max);
        state NegContactorCheck
          en:
          CTCd_iflt_NegCtrStuckOpen_fault=0;
          Timer.T1.Clear();
        (default) -> SlowCharge.Online.NegContactorDiagnose.NegContactorCheck
        SlowCharge.Online.NegContactorDiagnose.NegContactorDiag -> SlowCharge.Online.NegContactorDiagnose.NegContactorFault [order 2] : [(UAct3 > UAct1 *(1+ CTCc_pct_NegCtrDiagOpen)||...
            | UAct3 < UAct1 *(1- CTCc_pct_NegCtrDiagOpen))&&...
            | (CTCd_iflt_NegCtrStuckOpen_fault!=1)&&...
            | Timer.T1.Timeout==1]
        SlowCharge.Online.NegContactorDiagnose.NegContactorDiag -> SlowCharge.Online.NegContactorDiagnose.NegContactorCheck [order 1] : [UAct3 < UAct1 *(1+ CTCc_pct_NegCtrDiagCld)&&...
            | UAct3 >UAct1 *(1- CTCc_pct_NegCtrDiagCld)]
        SlowCharge.Online.NegContactorDiagnose.NegContactorCheck -> SlowCharge.Online.NegContactorDiagnose.NegContactorDiag : [UAct3 > UAct1 *(1+ CTCc_pct_NegCtrDiagOpen)||...
            | UAct3 < UAct1 *(1- CTCc_pct_NegCtrDiagOpen)]
    state Offline
      CTCd_enum_CtrSt = CTC_SlowChaOffline_St;
      CTCd_flg_PosCtrReq = 0;
      CTCd_flg_NegCtrReq = 0;
      CTCd_flg_PreCtrReq = 0;
      CTCd_flg_PosCtrSt = 0;
      CTCd_flg_NegCtrSt = 0;
      CTCd_flg_PreCtrSt = 0;
      ex:
      Timer.T3.Clear();
      Timer.T4.Clear();
      settings: description=$Author:Zhao XiangRi$
      state PreChargeAllow
        en:
        PreChargeAllow=1;
        du:
        Timer.T4.Run(CTCc_tm_PrecVoltAlow);
        ex:
        Timer.T4.Clear();
      state PreChargeProhibit
        en:
        PreChargeAllow=0;
        du:
        Timer.T3.Run(CTCc_tm_PrecVoltAlow);
        ex:
        Timer.T3.Clear();
      (default) -> SlowCharge.Offline.PreChargeProhibit
      SlowCharge.Offline.PreChargeProhibit -> SlowCharge.Offline.PreChargeAllow : [UAct4<(UAct1 * CTCc_pct_PrecVoltAllow)&&...
          | Timer.T3.Timeout ==1]
      SlowCharge.Offline.PreChargeAllow -> SlowCharge.Offline.PreChargeProhibit [order 1] : [UAct4>= (UAct1 * CTCc_pct_PrecVoltAllow)&&...
          | Timer.T4.Timeout ==1]
    state PreCharge
      en:
      CTCd_enum_CtrSt=CTC_SlowChaPreCharge_St;
      CTCd_flg_NegCtrSt=0;
      CTCd_flg_PreCtrSt=0;
      PreChargeFinish=0;
      du:
      CurrentGuard();
      ex:
      CTCd_iflt_NegCtrStuckOpen_fault=0;
      CTCd_iflt_PrecCurOver_fault=0;
      CTCd_iflt_PrecTmOver_fault=0;
      settings: description=$Author:Zhao XiangRi$
      state CurrentGuard [function]
        settings: description=$Author:Zhao XiangRi$
        (default) -> (junction 251)
        (junction 251) -> (junction 250) [order 3]
        (junction 251) -> (junction 252) [order 2] : [IAct<= CTCc_i_PrecCur_max && CTCd_iflt_PrecCurOver_fault != 0]
            | {CTCd_iflt_PrecCurOver_fault = 0;}
        (junction 251) -> (junction 253) [order 1] : [IAct>CTCc_i_PrecCur_max&& CTCd_iflt_PrecCurOver_fault!=1]
            | {CTCd_iflt_PrecCurOver_fault=1;}
      state NegContactorControl
        en:
        CTCd_flg_NegCtrSt=0;
        ex:
        Timer.T1.Clear();
        Timer.T2.Clear();
        CTCd_iflt_NegCtrStuckOpen_fault=0;
        settings: description=$Author:Zhao XiangRi$
        state CloseNegContactor
          en:
          CTCd_flg_NegCtrReq= 1;
          du:
          Timer.T1.Run(CTCc_tm_CtrClsCheckDly);
          Timer.T2.Run(CTCc_tm_CtrClsCheckDly_max);
        state CloseNegTimeOut
          en:
          CTCd_iflt_NegCtrStuckOpen_fault=1;
        state CloseNegContactorFinish
          en:
          CTCd_flg_NegCtrSt=1;
          CTCd_iflt_NegCtrStuckOpen_fault=0;
        (default) -> SlowCharge.PreCharge.NegContactorControl.CloseNegContactor
        SlowCharge.PreCharge.NegContactorControl.CloseNegContactor -> SlowCharge.PreCharge.NegContactorControl.CloseNegTimeOut [order 1] : [Timer.T2.Timeout==1&&CTCd_iflt_NegCtrStuckOpen_fault!=1]
        SlowCharge.PreCharge.NegContactorControl.CloseNegTimeOut -> SlowCharge.PreCharge.NegContactorControl.CloseNegContactor
        SlowCharge.PreCharge.NegContactorControl.CloseNegContactor -> SlowCharge.PreCharge.NegContactorControl.CloseNegContactorFinish [order 2] : [UAct3 <= UAct1 *(1+ CTCc_pct_NegCtrDiagCld)&&...
            | UAct3 >= UAct1 *(1- CTCc_pct_NegCtrDiagCld)&&...
            | Timer.T1.Timeout==1]
      state PreContactorControl
        en:
        CTCd_flg_PreCtrSt=0;
        ex:
        Timer.T1.Clear();
        settings: description=$Author:Zhao XiangRi$
        state ClosePreContactor
          en:
          CTCd_flg_PreCtrReq= 1;
          du:
          Timer.T1.Run(CTCc_tm_CtrClsCheckDly);
          ex:
          Timer.T1.Clear();
        state ClosePreContactorFinish
          en:
          CTCd_flg_PreCtrSt=1;
        (default) -> SlowCharge.PreCharge.PreContactorControl.ClosePreContactor
        SlowCharge.PreCharge.PreContactorControl.ClosePreContactor -> SlowCharge.PreCharge.PreContactorControl.ClosePreContactorFinish : [Timer.T1.Timeout==1]
      state PreChargeCheck
        du:
        Timer.T3.Run(CTCc_tm_PrecTm_max);
        ex:
        CTCd_iflt_PrecTmOver_fault= 0;
        Timer.T3.Clear();
        settings: description=$Author:Zhao XiangRi$
        state VoltageGradientCheck [function]
          settings: description=$Author:Zhao XiangRi$
          state Run(GradLimit,CountLimit) [function]
            (default) -> (junction 254)
            (junction 254) -> (junction 255) [order 1] : [GradLimitCorr == 0]
                | {GradLimitCorr = GradLimit * CTCc_tm_Tick_s;}
            (junction 255) -> (junction 254)
            (junction 254) -> (junction 256) [order 2] : {UGrad = UAct2 - UMem;}
            (junction 256) -> (junction 257) : {UMem = UAct2;}
            (junction 259) -> (junction 258) [order 1] : [Count >= CountLimit]
                | {Ok = 1;}
            (junction 257) -> (junction 259) [order 1] : [UGrad * CTCc_tm_Tick_s <= GradLimitCorr]
            (junction 259) -> (junction 260) [order 2] : {Count++;}
            (junction 257) -> (junction 260) [order 2] : {Ok = 0; Count = 0;}
          state Init [function]
            (default) -> (junction 261)
            (junction 261) -> (junction 262) : {UMem = 0; UGrad = 0; Count = 0; Ok = 0;...
                | GradLimitCorr = 0;}
        state PreChargeWait
          en:
          VoltageGradientCheck.Init();
          du:
          VoltageGradientCheck.Run(CTCc_v_PrecGradVolt,CTCc_cnt_PrecGradVoltDeb);
        state PrecDurMaxError
          en:
          CTCd_iflt_PrecTmOver_fault=1;
        state PreChargeFinish
          en:
          PreChargeFinish=1;
          CTCd_iflt_PrecTmOver_fault=0;
        (default) -> SlowCharge.PreCharge.PreChargeCheck.PreChargeWait
        SlowCharge.PreCharge.PreChargeCheck.PreChargeWait -> SlowCharge.PreCharge.PreChargeCheck.PrecDurMaxError [order 2] : [Timer.T3.Timeout ==1 &&CTCd_iflt_PrecTmOver_fault!= 1]
        SlowCharge.PreCharge.PreChargeCheck.PrecDurMaxError -> SlowCharge.PreCharge.PreChargeCheck.PreChargeWait
        SlowCharge.PreCharge.PreChargeCheck.PreChargeWait -> SlowCharge.PreCharge.PreChargeCheck.PreChargeFinish [order 1] : [UAct2>= (UAct1 * CTCc_pct_PrecTarVolt)&&...
            | (UAct1 - UAct2) <= CTCc_v_PrecTarVoltDif&&...
            | VoltageGradientCheck.Ok == 1&&...
            | CTCd_flg_PreCtrSt==1&&CTCd_flg_NegCtrSt==1]
      (default) -> SlowCharge.PreCharge.NegContactorControl
      SlowCharge.PreCharge.PreContactorControl.ClosePreContactorFinish -> SlowCharge.PreCharge.PreChargeCheck : [CTCd_flg_PreCtrSt==1]
      SlowCharge.PreCharge.NegContactorControl.CloseNegContactorFinish -> SlowCharge.PreCharge.PreContactorControl : [CTCd_flg_NegCtrSt==1]
    state Connect
      en:
      CTCd_enum_CtrSt=...
      CTC_SlowChaConnect_St;
      CTCd_flg_PosCtrSt=0;
      ConnectFinish=0;
      ex:
      CTCd_iflt_HVCnctCurOver_fault = 0;
      CTCd_iflt_HVCnctTmOver_fault=0;
      settings: description=$Author:Zhao XiangRi$
      state ConnectControl [parallel]
        settings: executionOrder=1  description=$Author:Zhao XiangRi$
        state PosContactorControl
          en:
          CTCd_flg_PosCtrSt=0;
          ex:
          CTCd_iflt_PosCtrStuckOpen_fault=0;
          settings: description=$Author:Zhao XiangRi$
          state ClosePosContactor
            en:
            CTCd_flg_PosCtrReq= 1;
            du:
            Timer.T1.Run(CTCc_tm_CtrClsCheckDly);
            Timer.T2.Run(CTCc_tm_CtrClsCheckDly_max);
            ex:
            Timer.T1.Clear();
            Timer.T2.Clear();
          state ClosePosTimeOut
            en:
            CTCd_iflt_PosCtrStuckOpen_fault=1;
          state ClosePosContactorFinish
            en:
            CTCd_flg_PosCtrSt=1;
            CTCd_iflt_PosCtrStuckOpen_fault=0;
          (default) -> SlowCharge.Connect.ConnectControl.PosContactorControl.ClosePosContactor
          SlowCharge.Connect.ConnectControl.PosContactorControl.ClosePosContactor -> SlowCharge.Connect.ConnectControl.PosContactorControl.ClosePosTimeOut [order 1] : [Timer.T2.Timeout==1&&CTCd_iflt_PosCtrStuckOpen_fault!=1]
          SlowCharge.Connect.ConnectControl.PosContactorControl.ClosePosTimeOut -> SlowCharge.Connect.ConnectControl.PosContactorControl.ClosePosContactor
          SlowCharge.Connect.ConnectControl.PosContactorControl.ClosePosContactor -> SlowCharge.Connect.ConnectControl.PosContactorControl.ClosePosContactorFinish [order 2] : [Timer.T1.Timeout==1&&...
              | UAct2<=UAct1 * (1+CTCc_pct_PosCtrDiagCld)&& ...
              | UAct2>= UAct1 *(1-CTCc_pct_PosCtrDiagCld) ]
        state PreContactorControl
          settings: description=$Author:Zhao XiangRi$
          state OpenPreContactor
            en:
            CTCd_flg_PreCtrReq= 0;
            du:
            Timer.T1.Run(CTCc_tm_CtrOpenCheckDly);
            ex:
            Timer.T1.Clear();
          state OpenPosContactorFinish
            en:
            CTCd_flg_PreCtrSt=0;
          SlowCharge.Connect.ConnectControl.PreContactorControl.OpenPreContactor -> SlowCharge.Connect.ConnectControl.PreContactorControl.OpenPosContactorFinish : [Timer.T1.Timeout==1]
          (default) -> SlowCharge.Connect.ConnectControl.PreContactorControl.OpenPreContactor
        (default) -> SlowCharge.Connect.ConnectControl.PosContactorControl
        SlowCharge.Connect.ConnectControl.PosContactorControl.ClosePosContactorFinish -> SlowCharge.Connect.ConnectControl.PreContactorControl : [CTCd_flg_PosCtrSt==1]
      state ConnectCheck [parallel]
        du:
        CurrentGuard();
        Timer.T3.Run(CTCc_tm_HVCnctTm_max);
        ex:
        Timer.T3.Clear();
        settings: executionOrder=2  description=$Author:Zhao XiangRi$
        state CurrentGuard [function]
          settings: description=$Author:Zhao XiangRi$
          (junction 264) -> (junction 239) [order 2] : [IAct<= CTCc_i_HVCnctCur_max&& CTCd_iflt_HVCnctCurOver_fault != 0]
              | {CTCd_iflt_HVCnctCurOver_fault = 0;}
          (junction 264) -> (junction 263) [order 3]
          (default) -> (junction 264)
          (junction 264) -> (junction 238) [order 1] : [IAct> CTCc_i_HVCnctCur_max&& CTCd_iflt_HVCnctCurOver_fault != 1]
              | {CTCd_iflt_HVCnctCurOver_fault = 1;}
        state ConnectWait
        state CnctDurMaxError
          en:
          CTCd_iflt_HVCnctTmOver_fault=1;
        state ConnectFinish
          en:
          ConnectFinish=1;
          CTCd_iflt_HVCnctTmOver_fault=0;
        (default) -> SlowCharge.Connect.ConnectCheck.ConnectWait
        SlowCharge.Connect.ConnectCheck.ConnectWait -> SlowCharge.Connect.ConnectCheck.ConnectFinish [order 1] : [UAct2 >= (UAct1 * CTCc_pct_HVCnctTarVolt)&&...
            |  CTCd_flg_PosCtrSt==1&&...
            | CTCd_flg_PreCtrSt==0]
        SlowCharge.Connect.ConnectCheck.ConnectWait -> SlowCharge.Connect.ConnectCheck.CnctDurMaxError [order 2] : [Timer.T3.Timeout ==1&&CTCd_iflt_HVCnctTmOver_fault!=1]
        SlowCharge.Connect.ConnectCheck.CnctDurMaxError -> SlowCharge.Connect.ConnectCheck.ConnectWait
    state EmergencyDisconnect
      en:
      CTCd_enum_CtrSt=...
      CTC_DriveEmgyDcnct_St;
      DcnctEmcyFinish = 0;
      settings: description=$Author:Zhao XiangRi$
      state EmcyDisconnectControl [parallel]
        en:
        CTCd_flg_PosCtrReq= 0;
        CTCd_flg_NegCtrReq= 0;
        CTCd_flg_PreCtrReq= 0;
        DcnctEmcyCtlFinish = 1;
        settings: executionOrder=1  description=$Author:Zhao XiangRi$
      state EmcyDisconnectCheck [parallel]
        du:
        Timer.T1.Run(CTCc_tm_HVEmcyDcnctTm_max);
        ex:
        Timer.T1.Clear();
        settings: executionOrder=2  description=$Author:Zhao XiangRi$
        state DisconnectWait
        state DisconnectComplete
          DcnctEmcyFinish = 1;
        state DisconnectTimeoutError
          en:
          CTCd_iflt_HVEmcyDcnctTmOver_fault = 1;
          ex:
          CTCd_iflt_HVEmcyDcnctTmOver_fault = 0;
        SlowCharge.EmergencyDisconnect.EmcyDisconnectCheck.DisconnectTimeoutError -> SlowCharge.EmergencyDisconnect.EmcyDisconnectCheck.DisconnectComplete : [DcnctEmcyCtlFinish==1 &&...
            | (UAct2>= UAct1 * (1 +CTCc_pct_HVDcnctTarVolt) ||UAct2<= UAct1 * (1 - CTCc_pct_HVDcnctTarVolt))]
            | {CTCd_flg_PosCtrSt=0;CTCd_flg_NegCtrSt=0;CTCd_flg_PreCtrSt=0;}
        SlowCharge.EmergencyDisconnect.EmcyDisconnectCheck.DisconnectWait -> SlowCharge.EmergencyDisconnect.EmcyDisconnectCheck.DisconnectComplete [order 2] : [DcnctEmcyCtlFinish==1 &&IAct<= CTCc_i_HVDcnctCur_max &&...
            | (UAct2>= UAct1 * (1 + CTCc_pct_HVDcnctTarVolt) ||UAct2<= UAct1 * (1 - CTCc_pct_HVDcnctTarVolt))]
            | {CTCd_flg_PosCtrSt=0;CTCd_flg_NegCtrSt=0;CTCd_flg_PreCtrSt=0;}
        (default) -> SlowCharge.EmergencyDisconnect.EmcyDisconnectCheck.DisconnectWait
        SlowCharge.EmergencyDisconnect.EmcyDisconnectCheck.DisconnectWait -> SlowCharge.EmergencyDisconnect.EmcyDisconnectCheck.DisconnectTimeoutError [order 1] : [Timer.T1.Timeout == 1]
    (default) -> SlowCharge.Offline
    (junction 242) -> SlowCharge.Offline
    (junction 248) -> (junction 242)
    (junction 243) -> SlowCharge.Offline
    SlowCharge.PreCharge -> (junction 244) : [CTCd_iflt_NegCtrStuckOpen_fault==1||...
        | CTCd_iflt_PrecCurOver_fault==1||...
        | CTCd_iflt_PrecTmOver_fault==1]
    (junction 244) -> (junction 245)
    SlowCharge.Offline.PreChargeAllow -> SlowCharge.PreCharge [order 2] : [DEMd_enum_CtrCmd==CTC_SlowChaOnline_CtrCmd&&...
        | BSCd_enum_BCUSt==BCU_SlowCharge_St&&...
        | PreChargeAllow==1]
    SlowCharge.Disconnect.DisConnectCheck.DisConnectFinish -> (junction 248) : [DisConnectFinish==1]
    SlowCharge.Connect.ConnectCheck.ConnectFinish -> SlowCharge.Online : [ConnectFinish==1]
    SlowCharge.Connect -> (junction 245) : [CTCd_iflt_HVCnctCurOver_fault==1||...
        | CTCd_iflt_HVCnctTmOver_fault==1]
    SlowCharge.PreCharge.PreChargeCheck.PreChargeFinish -> SlowCharge.Connect : [PreChargeFinish==1]
    (junction 245) -> (junction 246)
    SlowCharge.EmergencyDisconnect.EmcyDisconnectCheck.DisconnectComplete -> (junction 243) : [DcnctEmcyFinish == 1]
    (junction 246) -> SlowCharge.EmergencyDisconnect
    (junction 247) -> (junction 246)
    SlowCharge.Online -> SlowCharge.Disconnect : [DEMd_enum_CtrCmd==CTC_SlowChaOffline_CtrCmd||...
        | DEMd_enum_CtrCmd~=CTC_SlowChaOnline_CtrCmd]
    (junction 249) -> (junction 247)
    SlowCharge.Disconnect -> (junction 249) : [CTCd_iflt_HVDcnctTmOver_fault==1]
  DefaultOffline -> Service [order 4] : [BSCd_enum_BCUSt==BCU_Service_St]
  Service -> DefaultOffline : [IPTd_flg_ServSt==0&&...
      | CTCd_enum_CtrSt ==CTC_ServiceOffline_St]
  (default) -> DefaultOffline
  SlowCharge -> DefaultOffline : [IPTd_flg_SlowChaCnctSt==0&&...
      | CTCd_enum_CtrSt == CTC_SlowChaOffline_St]
  Drive -> DefaultOffline : [IPTd_flg_KL15==0&&...
      | CTCd_enum_CtrSt==CTC_DriveOffline_St]
  FastCharge -> DefaultOffline : [IPTd_flg_FastChaCnctSt==0&&...
      | CTCd_enum_CtrSt == CTC_FastChaOffline_St]
  DefaultOffline -> SlowCharge [order 3] : [BSCd_enum_BCUSt==BCU_SlowCharge_St]
  DefaultOffline -> FastCharge [order 1] : [BSCd_enum_BCUSt==BCU_FastCharge_St]
  DefaultOffline -> Drive [order 2] : [BSCd_enum_BCUSt==BCU_Drive_St]
  data: Timeout local boolean; TimeLimit local single; TimeTicks local single; Init local boolean; Limit function_input single; Timeout local boolean; TimeLimit local single; TimeTicks local single; Init local boolean; Limit function_input single; Timeout local boolean; TimeLimit local single; TimeTicks local single; Init local boolean; Limit function_input single; Timeout local boolean; TimeLimit local single; TimeTicks local single; Init local boolean; Limit function_input single; UGrad local single; UMem local single; Count local uint8; Ok local boolean; GradLimitCorr local single; GradLimit function_input single; CountLimit function_input uint8; DcnctEmcyCtlFinish local boolean; UGrad local single; UMem local single; Count local uint8; Ok local boolean; GradLimitCorr local single; GradLimit function_input single; CountLimit function_input uint8; DcnctEmcyCtlFinish local boolean; BSCd_enum_BCUSt input double; DEMd_enum_CtrCmd input uint8; IPTd_flg_KL15 input boolean; IPTd_flg_SlowChaCnctSt input boolean; IPTd_flg_FastChaCnctSt input boolean; IPTd_flg_ServSt input boolean; CTCd_enum_CtrSt output uint8; CTCd_flg_PosCtrSt output boolean; CTCd_flg_NegCtrSt output boolean; CTCd_flg_PreCtrSt output boolean; CTCd_flg_FastChaCtrSt output boolean; CTCd_flg_SlowChaCtrSt output boolean; CTCd_flg_PosCtrReq output boolean; CTCd_flg_NegCtrReq output boolean; CTCd_flg_PreCtrReq output boolean; CTCd_flg_FastChaCtrReq output boolean; CTCd_flg_SlowChaCtrReq output boolean; IPTd_enum_ServCmd input uint8; UAct1 input single; UAct2 input single; UAct3 input single; UAct4 input single; IAct input boolean; CTCd_iflt_PrecTmOver_fault output boolean; CTCc_tm_Tick_s input single; CTCc_tm_CtrClsCheckDly input single; CTCc_tm_CtrClsCheckDly_max input single; CTCc_tm_CtrOpenCheckDly input single; CTCc_tm_CtrOpenCheck_max input single; CTCd_iflt_HVCnctTmOver_fault output boolean; CTCd_iflt_HVDcncWaitTmOver_fault output boolean; CTCd_iflt_HVDcnctTmOver_fault output boolean; CTCd_iflt_HVEmcyDcnctTmOver_fault output boolean; CTCd_iflt_PrecCurOver_fault output boolean; CTCd_iflt_HVCnctCurOver_fault output boolean; PreChargeFinish local boolean; ShutoffFinish local boolean; DisConnectFinish local boolean; DcnctEmcyFinish local boolean; CTCc_tm_PrecTm_max input single; CTCc_tm_HVCnctTm_max input single; CTCc_tm_HVDcnctWaitTm_max input single; CTCc_tm_HVDcnctWaitTm input single; CTCc_tm_HVDcnctTm_max input single; CTCc_tm_HVEmcyDcnctTm_max input single; CTCc_i_PrecCur_max input single; CTCc_i_HVCnctCur_max input single; CTCc_i_HVDcncWaitCur_max input single; CTCc_i_HVDcnctCur_max input double; CTCc_pct_PrecTarVolt input single; CTCc_v_PrecTarVoltDif input single; CTCc_v_PrecGradVolt input uint8; CTCc_cnt_PrecGradVoltDeb input single; CTCc_pct_HVCnctTarVolt input single; CTCc_pct_HVDcnctTarVolt input single; CTCd_iflt_NegCtrStuckOpen_fault output boolean; CTCd_iflt_NegCtrStuckCld_fault output boolean; CTCd_iflt_PosCtrStuckOpen_fault output boolean; CTCd_iflt_PosCtrStuckCld_fault output boolean; ConnectFinish local boolean; CTCc_pct_NegCtrDiagCld input double; CTCc_pct_NegCtrDiagOpen input double; CTCc_pct_PosCtrDiagCld input double; CTCc_pct_PosCtrDiagOpen input double; CTC_DrivePrecharge_St parameter uint8; CTC_DriveConnect_St parameter uint8; CTC_DriveDisconnect_St parameter uint8; CTC_DriveEmgyDcnct_St parameter uint8; CTC_DriveOffline_St parameter uint8; CTC_DriveOnline_St parameter uint8; CTC_FastChaOffline_St parameter uint8; CTC_FastChaConnect_St parameter uint8; BCU_Drive_St parameter uint8; BCU_FastCharge_St parameter uint8; BCU_SlowCharge_St parameter uint8; BCU_Service_St parameter uint8; CTC_FastChaOnline_St parameter uint8; CTC_FastChaDisconnect_St parameter uint8; CTC_SlowChaConnect_St parameter uint8; CTC_SlowChaOffline_St parameter uint8; CTC_SlowChaDisconnect_St parameter uint8; CTC_SlowChaOnline_St parameter uint8; CTC_DefaultOffline_St parameter uint8; CTC_OpenNegCtr_SerCmd parameter uint8; CTC_CloseNegCtr_SerCmd parameter uint8; CTC_OpenPosCtr_SerCmd parameter uint8; CTC_ClosePosCtr_SerCmd parameter uint8; CTC_OpenPreCtr_SerCmd parameter uint8; CTC_ClosePreCtr_SerCmd parameter uint8; CTC_OpenFastChaCtr_SerCmd parameter uint8; CTC_CloseFastChaCtr_SerCmd parameter uint8; CTC_OpenSlowChaCtr_SerCmd parameter uint8; CTC_CloseSlowChaCtr_SerCmd parameter uint8; CTC_ServiceOffline_St parameter uint8; CTC_ServiceOnline_St parameter uint8; CTC_FastChaOffline_CtrCmd parameter uint8; CTC_FastChaOnline_CtrCmd parameter uint8; CTC_DriveShutoff_St parameter uint8; CTC_SlowChaOffline_CtrCmd parameter uint8; CTC_SlowChaOnline_CtrCmd parameter uint8; FastChaConnectFinish local boolean; FastChaDisconnectFinish local boolean; SlowChaConnectFinish local boolean; SlowChaDisconnectFinish local boolean; CTC_DriveEmgyDcnct_CtrCmd parameter uint8; CTC_DriveOffline_CtrCmd parameter uint8; CTC_DriveOnline_CtrCmd parameter uint8; PreChargeAllow local boolean; CTCc_pct_PrecVoltAllow input double; CTCc_tm_PrecVoltAlow input double; Lock local boolean; CTC_SlowChaPreCharge_St parameter double
  data UAct2 settings: description=Actual Voltage 1: High Voltage + after battery and before contactor (Pack Voltage)
  data UAct3 settings: description=Actual Voltage 2: High Voltage + after battery and after contactor
  data UAct4 settings: description=Actual Voltage 2: High Voltage + after battery and after contactor
  data IAct settings: description=Actual Voltage 2: High Voltage + after battery and after contactor
